simulink model "exsim3modelPart2"  (R2018b)
settings: Solver=VariableStepAuto  StartTime=0.0  StopTime=10.0  RelTol=1e-3
values from neighbouring files (symbols this model uses):
  nb = eval(solutionKb(2))    [exsim3.m]
  Ts = 0.2    [exsim3.m]
libraries: simulink x1
settings Model: Creator=rafael  LastModifiedBy=rafael

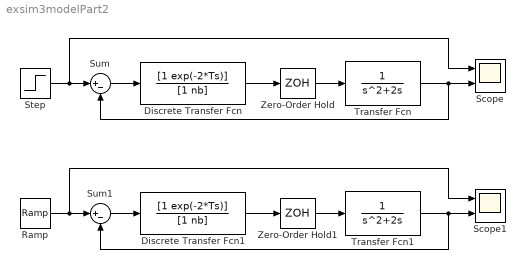
== system exsim3modelPart2 ==
  Discrete Transfer Fcn : DiscreteTransferFcn  Numerator=[1 exp(-2*Ts)]  Denominator=[1 nb]  SampleTime=Ts
  Discrete Transfer Fcn1 : DiscreteTransferFcn  Numerator=[1 exp(-2*Ts)]  Denominator=[1 nb]  SampleTime=Ts
  Ramp : simulink/Sources/Ramp  slope=1  start=0  InitialOutput=0
  Scope : Scope  NumInputPorts=2
  Scope1 : Scope  NumInputPorts=2
  Step : Step  SampleTime=0
  Sum : Sum  Inputs=|+-
  Sum1 : Sum  Inputs=|+-
  Transfer Fcn : TransferFcn  Denominator=[1 2 0]
  Transfer Fcn1 : TransferFcn  Denominator=[1 2 0]
  Zero-Order Hold : ZeroOrderHold  SampleTime=Ts
  Zero-Order Hold1 : ZeroOrderHold  SampleTime=Ts
  wires:
  Zero-Order Hold/1 -> Transfer Fcn/1
  Discrete Transfer Fcn/1 -> Zero-Order Hold/1
  Sum/1 -> Discrete Transfer Fcn/1
  Transfer Fcn/1 -> Sum/2, Scope/2
  Step/1 -> Scope/1, Sum/1
  Ramp/1 -> Scope1/1, Sum1/1
  Discrete Transfer Fcn1/1 -> Zero-Order Hold1/1
  Transfer Fcn1/1 -> Sum1/2, Scope1/2
  Sum1/1 -> Discrete Transfer Fcn1/1
  Zero-Order Hold1/1 -> Transfer Fcn1/1
